simulink model "lista1_questao1"  (R2014b)
settings: Solver=ode45  StartTime=0.0  StopTime=20  RelTol=1e-3
libraries: cstblocks x2
settings Model: Creator=Danilo  LastModifiedBy=Danilo

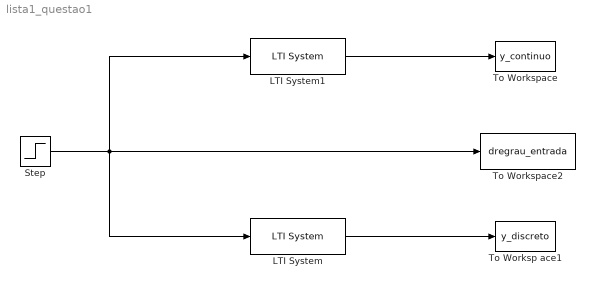
== system lista1_questao1 ==
  LTI System : cstblocks/LTI System  sys=Hd  IC=[]
  LTI System1 : cstblocks/LTI System  sys=H  IC=[]
  Step : Step  Before=0.1  SampleTime=0
  To Worksp ace1 : ToWorkspace  VariableName=y_discreto  SaveFormat=Timeseries  SampleTime=-1
  To Workspace : ToWorkspace  VariableName=y_continuo  SaveFormat=Timeseries  SampleTime=-1
  To Workspace2 : ToWorkspace  VariableName=dregrau_entrada  SaveFormat=Timeseries  SampleTime=-1
  wires:
  Step/1 -> LTI System/1, LTI System1/1, To Workspace2/1
  LTI System/1 -> To Worksp ace1/1
  LTI System1/1 -> To Workspace/1
